simulink model "case5"  (R2024b)
settings: Solver=FixedStepAuto  StartTime=0  StopTime=1  FixedStep=1e-7  RelTol=1e-3
values from neighbouring files (symbols this model uses):
  SG_D_1_D = 0.01056    [IEEE9_case_parameters.m]    (also in case1_parameters.m; case2_parameters.m; case3_parameters.m; case4_parameters.m)
  SG_D_1_EnableSaturation = 0    [IEEE9_case_parameters.m]    (also in case1_parameters.m; case2_parameters.m; case3_parameters.m; case4_parameters.m)
  SG_D_1_f0 = 60    [IEEE9_case_parameters.m]    (also in case1_parameters.m; case2_parameters.m; case3_parameters.m; case4_parameters.m)
  SG_D_1_H = 7.5    [IEEE9_case_parameters.m]    (also in case1_parameters.m; case2_parameters.m; case3_parameters.m; case4_parameters.m)
  SG_D_1_K_A = 20    [IEEE9_case_parameters.m]    (also in case1_parameters.m; case2_parameters.m; case3_parameters.m; case4_parameters.m)
  SG_D_1_K_E = 1.000000e+1    (= 10)    [IEEE9_case_parameters.m]    (also in case1_parameters.m; case2_parameters.m; case3_parameters.m; case4_parameters.m)
  SG_D_1_K_F = 2.363    [IEEE9_case_parameters.m]    (also in case1_parameters.m; case2_parameters.m; case3_parameters.m; case4_parameters.m)
  SG_D_1_K_s = 0.5    [IEEE9_case_parameters.m]    (also in case1_parameters.m = 5; case2_parameters.m = 5; case3_parameters.m = 5; case4_parameters.m = 5)
  SG_D_1_R_a = 0.001088    [IEEE9_case_parameters.m]    (also in case1_parameters.m; case2_parameters.m; case3_parameters.m; case4_parameters.m)
  SG_D_1_S_A = 1    [IEEE9_case_parameters.m]    (also in case1_parameters.m; case2_parameters.m; case3_parameters.m; case4_parameters.m)
  SG_D_1_S_B = 0.103    [IEEE9_case_parameters.m]    (also in case1_parameters.m; case2_parameters.m; case3_parameters.m; case4_parameters.m)
  SG_D_1_S_N = 10.659857    [IEEE9_case_parameters.m]    (also in case1_parameters.m; case2_parameters.m; case3_parameters.m; case4_parameters.m)
  SG_D_1_SpeedPara = 200    [IEEE9_case_parameters.m]    (also in case1_parameters.m; case2_parameters.m; case3_parameters.m; case4_parameters.m)
  SG_D_1_T_0 = 0.720173    [IEEE9_case_parameters.m]    (also in case1_parameters.m = 0.755522; case2_parameters.m = 0.808931; case3_parameters.m = 0.869402; case4_parameters.m = 0.729316)
  SG_D_1_T_1 = 0.3    [IEEE9_case_parameters.m]    (also in case1_parameters.m; case2_parameters.m; case3_parameters.m; case4_parameters.m)
  SG_D_1_T_2 = 0.05    [IEEE9_case_parameters.m]    (also in case1_parameters.m; case2_parameters.m; case3_parameters.m; case4_parameters.m)
  SG_D_1_T_3 = 0.02    [IEEE9_case_parameters.m]    (also in case1_parameters.m; case2_parameters.m; case3_parameters.m; case4_parameters.m)
  SG_D_1_T_4 = 0.005    [IEEE9_case_parameters.m]    (also in case1_parameters.m; case2_parameters.m; case3_parameters.m; case4_parameters.m)
  SG_D_1_T_A = 0.02    [IEEE9_case_parameters.m]    (also in case1_parameters.m; case2_parameters.m; case3_parameters.m; case4_parameters.m)
  SG_D_1_T_dd = 8.000000e+0    (= 8)    [IEEE9_case_parameters.m]    (also in case1_parameters.m; case2_parameters.m; case3_parameters.m; case4_parameters.m)
  SG_D_1_T_ddd = 0.04    [IEEE9_case_parameters.m]    (also in case1_parameters.m; case2_parameters.m; case3_parameters.m; case4_parameters.m)
  SG_D_1_T_E = 0.314    [IEEE9_case_parameters.m]    (also in case1_parameters.m; case2_parameters.m; case3_parameters.m; case4_parameters.m)
  SG_D_1_T_F = 0.35    [IEEE9_case_parameters.m]    (also in case1_parameters.m; case2_parameters.m; case3_parameters.m; case4_parameters.m)
  SG_D_1_T_qd = 0.8    [IEEE9_case_parameters.m]    (also in case1_parameters.m; case2_parameters.m; case3_parameters.m; case4_parameters.m)
  SG_D_1_T_qdd = 0.02    [IEEE9_case_parameters.m]    (also in case1_parameters.m; case2_parameters.m; case3_parameters.m; case4_parameters.m)
  SG_D_1_T_speed = 0.1    [IEEE9_case_parameters.m]    (also in case1_parameters.m = 200; case2_parameters.m = 200; case3_parameters.m = 200; case4_parameters.m = 200)
  SG_D_1_T_w = 0.5    [IEEE9_case_parameters.m]    (also in case1_parameters.m; case2_parameters.m; case3_parameters.m; case4_parameters.m)
  SG_D_1_V_ref = 1.990276    [IEEE9_case_parameters.m]    (also in case1_parameters.m = 2.042296; case2_parameters.m = 2.051388; case3_parameters.m = 2.089584; case4_parameters.m = 2.01845)
  SG_D_1_w_ref = 376.991118    [IEEE9_case_parameters.m]    (also in case1_parameters.m; case2_parameters.m; case3_parameters.m; case4_parameters.m)
  SG_D_1_wb = 6.000000e+1    (= 60)    [IEEE9_case_parameters.m]    (also in case1_parameters.m; case2_parameters.m; case3_parameters.m; case4_parameters.m)
  SG_D_1_x_d = 1.9    [IEEE9_case_parameters.m]    (also in case1_parameters.m; case2_parameters.m; case3_parameters.m; case4_parameters.m)
  SG_D_1_x_dd = 0.302    [IEEE9_case_parameters.m]    (also in case1_parameters.m; case2_parameters.m; case3_parameters.m; case4_parameters.m)
  SG_D_1_x_ddd = 0.204    [IEEE9_case_parameters.m]    (also in case1_parameters.m; case2_parameters.m; case3_parameters.m; case4_parameters.m)
  SG_D_1_x_l = 0.05    [IEEE9_case_parameters.m]    (also in case1_parameters.m; case2_parameters.m; case3_parameters.m; case4_parameters.m)
  SG_D_1_x_q = 1.3    [IEEE9_case_parameters.m]    (also in case1_parameters.m; case2_parameters.m; case3_parameters.m; case4_parameters.m)
  SG_D_1_x_qd = 0.5    [IEEE9_case_parameters.m]    (also in case1_parameters.m; case2_parameters.m; case3_parameters.m; case4_parameters.m)
  SG_D_1_x_qdd = 0.3    [IEEE9_case_parameters.m]    (also in case1_parameters.m; case2_parameters.m; case3_parameters.m; case4_parameters.m)
  SG_D_2_D = 0.02    [IEEE9_case_parameters.m]    (also in case1_parameters.m; case2_parameters.m; case3_parameters.m; case4_parameters.m)
  SG_D_2_EnableSaturation = 0    [IEEE9_case_parameters.m]    (also in case1_parameters.m; case2_parameters.m; case3_parameters.m; case4_parameters.m)
  SG_D_2_f0 = 60    [IEEE9_case_parameters.m]    (also in case1_parameters.m; case2_parameters.m; case3_parameters.m; case4_parameters.m)
  SG_D_2_H = 8.000000e+0    (= 8)    [IEEE9_case_parameters.m]    (also in case1_parameters.m; case2_parameters.m; case3_parameters.m; case4_parameters.m)
  SG_D_2_K_A = 20    [IEEE9_case_parameters.m]    (also in case1_parameters.m; case2_parameters.m; case3_parameters.m; case4_parameters.m)
  SG_D_2_K_E = 1.000000e+1    (= 10)    [IEEE9_case_parameters.m]    (also in case1_parameters.m; case2_parameters.m; case3_parameters.m; case4_parameters.m)
  SG_D_2_K_F = 2.363    [IEEE9_case_parameters.m]    (also in case1_parameters.m; case2_parameters.m; case3_parameters.m; case4_parameters.m)
  SG_D_2_K_s = 0.5    [IEEE9_case_parameters.m]    (also in case1_parameters.m = 4; case2_parameters.m = 4; case3_parameters.m = 4; case4_parameters.m = 4)
  SG_D_2_R_a = 0.001088    [IEEE9_case_parameters.m]    (also in case1_parameters.m; case2_parameters.m; case3_parameters.m; case4_parameters.m)
  SG_D_2_S_A = 1    [IEEE9_case_parameters.m]    (also in case1_parameters.m; case2_parameters.m; case3_parameters.m; case4_parameters.m)
  SG_D_2_S_B = 0.103    [IEEE9_case_parameters.m]    (also in case1_parameters.m; case2_parameters.m; case3_parameters.m; case4_parameters.m)
  SG_D_2_S_N = 10.659857    [IEEE9_case_parameters.m]    (also in case1_parameters.m; case2_parameters.m; case3_parameters.m; case4_parameters.m)
  SG_D_2_SpeedPara = 200    [IEEE9_case_parameters.m]    (also in case1_parameters.m; case2_parameters.m; case3_parameters.m; case4_parameters.m)
  SG_D_2_T_0 = 1.632913    [IEEE9_case_parameters.m]    (also in case1_parameters.m = 1.632925; case2_parameters.m = 1.632915; case3_parameters.m = 1.632914; case4_parameters.m = 1.632927)
  SG_D_2_T_1 = 0.2    [IEEE9_case_parameters.m]    (also in case1_parameters.m; case2_parameters.m; case3_parameters.m; case4_parameters.m)
  SG_D_2_T_2 = 0.05    [IEEE9_case_parameters.m]    (also in case1_parameters.m; case2_parameters.m; case3_parameters.m; case4_parameters.m)
  SG_D_2_T_3 = 0.02    [IEEE9_case_parameters.m]    (also in case1_parameters.m; case2_parameters.m; case3_parameters.m; case4_parameters.m)
  SG_D_2_T_4 = 0.005    [IEEE9_case_parameters.m]    (also in case1_parameters.m; case2_parameters.m; case3_parameters.m; case4_parameters.m)
  SG_D_2_T_A = 0.02    [IEEE9_case_parameters.m]    (also in case1_parameters.m; case2_parameters.m; case3_parameters.m; case4_parameters.m)
  SG_D_2_T_dd = 7.9    [IEEE9_case_parameters.m]    (also in case1_parameters.m; case2_parameters.m; case3_parameters.m; case4_parameters.m)
  SG_D_2_T_ddd = 0.04    [IEEE9_case_parameters.m]    (also in case1_parameters.m; case2_parameters.m; case3_parameters.m; case4_parameters.m)
  SG_D_2_T_E = 0.314    [IEEE9_case_parameters.m]    (also in case1_parameters.m; case2_parameters.m; case3_parameters.m; case4_parameters.m)
  SG_D_2_T_F = 0.35    [IEEE9_case_parameters.m]    (also in case1_parameters.m; case2_parameters.m; case3_parameters.m; case4_parameters.m)
  SG_D_2_T_qd = 0.8    [IEEE9_case_parameters.m]    (also in case1_parameters.m; case2_parameters.m; case3_parameters.m; case4_parameters.m)
  SG_D_2_T_qdd = 0.015    [IEEE9_case_parameters.m]    (also in case1_parameters.m; case2_parameters.m; case3_parameters.m; case4_parameters.m)
  SG_D_2_T_speed = 0.1    [IEEE9_case_parameters.m]    (also in case1_parameters.m = 150; case2_parameters.m = 150; case3_parameters.m = 150; case4_parameters.m = 150)
  SG_D_2_T_w = 0.35    [IEEE9_case_parameters.m]    (also in case1_parameters.m; case2_parameters.m; case3_parameters.m; case4_parameters.m)
  SG_D_2_V_ref = 2.58547    [IEEE9_case_parameters.m]    (also in case1_parameters.m = 2.597896; case2_parameters.m = 2.587136; case3_parameters.m = 2.586042; case4_parameters.m = 2.599679)
  SG_D_2_w_ref = 376.991118    [IEEE9_case_parameters.m]    (also in case1_parameters.m; case2_parameters.m; case3_parameters.m; case4_parameters.m)
  SG_D_2_wb = 6.000000e+1    (= 60)    [IEEE9_case_parameters.m]    (also in case1_parameters.m; case2_parameters.m; case3_parameters.m; case4_parameters.m)
  SG_D_2_x_d = 1.8    [IEEE9_case_parameters.m]    (also in case1_parameters.m; case2_parameters.m; case3_parameters.m; case4_parameters.m)
  SG_D_2_x_dd = 0.302    [IEEE9_case_parameters.m]    (also in case1_parameters.m; case2_parameters.m; case3_parameters.m; case4_parameters.m)
  SG_D_2_x_ddd = 0.204    [IEEE9_case_parameters.m]    (also in case1_parameters.m; case2_parameters.m; case3_parameters.m; case4_parameters.m)
  SG_D_2_x_l = 0.05    [IEEE9_case_parameters.m]    (also in case1_parameters.m; case2_parameters.m; case3_parameters.m; case4_parameters.m)
  SG_D_2_x_q = 1.25    [IEEE9_case_parameters.m]    (also in case1_parameters.m; case2_parameters.m; case3_parameters.m; case4_parameters.m)
  SG_D_2_x_qd = 0.5    [IEEE9_case_parameters.m]    (also in case1_parameters.m; case2_parameters.m; case3_parameters.m; case4_parameters.m)
  SG_D_2_x_qdd = 0.3    [IEEE9_case_parameters.m]    (also in case1_parameters.m; case2_parameters.m; case3_parameters.m; case4_parameters.m)
  SG_D_3_D = 0.02    [IEEE9_case_parameters.m]    (also in case1_parameters.m; case2_parameters.m; case3_parameters.m; case4_parameters.m)
  SG_D_3_EnableSaturation = 0    [IEEE9_case_parameters.m]    (also in case1_parameters.m; case2_parameters.m; case3_parameters.m; case4_parameters.m)
  SG_D_3_f0 = 60    [IEEE9_case_parameters.m]    (also in case1_parameters.m; case2_parameters.m; case3_parameters.m; case4_parameters.m)
  SG_D_3_H = 7.7    [IEEE9_case_parameters.m]    (also in case1_parameters.m; case2_parameters.m; case3_parameters.m; case4_parameters.m)
  SG_D_3_K_A = 20    [IEEE9_case_parameters.m]    (also in case1_parameters.m; case2_parameters.m; case3_parameters.m; case4_parameters.m)
  SG_D_3_K_E = 1.000000e+1    (= 10)    [IEEE9_case_parameters.m]    (also in case1_parameters.m; case2_parameters.m; case3_parameters.m; case4_parameters.m)
  SG_D_3_K_F = 2.363    [IEEE9_case_parameters.m]    (also in case1_parameters.m; case2_parameters.m; case3_parameters.m; case4_parameters.m)
  SG_D_3_K_s = 0.2    [IEEE9_case_parameters.m]    (also in case1_parameters.m = 2; case2_parameters.m = 2; case3_parameters.m = 2; case4_parameters.m = 2)
  SG_D_3_R_a = 0.001088    [IEEE9_case_parameters.m]    (also in case1_parameters.m; case2_parameters.m; case3_parameters.m; case4_parameters.m)
  SG_D_3_S_A = 1    [IEEE9_case_parameters.m]    (also in case1_parameters.m; case2_parameters.m; case3_parameters.m; case4_parameters.m)
  SG_D_3_S_B = 0.103    [IEEE9_case_parameters.m]    (also in case1_parameters.m; case2_parameters.m; case3_parameters.m; case4_parameters.m)
  SG_D_3_S_N = 10.659857    [IEEE9_case_parameters.m]    (also in case1_parameters.m; case2_parameters.m; case3_parameters.m; case4_parameters.m)
  SG_D_3_SpeedPara = 200    [IEEE9_case_parameters.m]    (also in case1_parameters.m; case2_parameters.m; case3_parameters.m; case4_parameters.m)
  SG_D_3_T_0 = 0.850788    [IEEE9_case_parameters.m]    (also in case1_parameters.m = 0.850786; case2_parameters.m = 0.850787; case3_parameters.m; case4_parameters.m = 0.850786)
  SG_D_3_T_1 = 0.2    [IEEE9_case_parameters.m]    (also in case1_parameters.m; case2_parameters.m; case3_parameters.m; case4_parameters.m)
  SG_D_3_T_2 = 0.05    [IEEE9_case_parameters.m]    (also in case1_parameters.m; case2_parameters.m; case3_parameters.m; case4_parameters.m)
  SG_D_3_T_3 = 0.02    [IEEE9_case_parameters.m]    (also in case1_parameters.m; case2_parameters.m; case3_parameters.m; case4_parameters.m)
  SG_D_3_T_4 = 0.005    [IEEE9_case_parameters.m]    (also in case1_parameters.m; case2_parameters.m; case3_parameters.m; case4_parameters.m)
  SG_D_3_T_A = 0.02    [IEEE9_case_parameters.m]    (also in case1_parameters.m; case2_parameters.m; case3_parameters.m; case4_parameters.m)
  SG_D_3_T_dd = 8.1    [IEEE9_case_parameters.m]    (also in case1_parameters.m; case2_parameters.m; case3_parameters.m; case4_parameters.m)
  SG_D_3_T_ddd = 0.04    [IEEE9_case_parameters.m]    (also in case1_parameters.m; case2_parameters.m; case3_parameters.m; case4_parameters.m)
  SG_D_3_T_E = 0.314    [IEEE9_case_parameters.m]    (also in case1_parameters.m; case2_parameters.m; case3_parameters.m; case4_parameters.m)
  SG_D_3_T_F = 0.35    [IEEE9_case_parameters.m]    (also in case1_parameters.m; case2_parameters.m; case3_parameters.m; case4_parameters.m)
  SG_D_3_T_qd = 0.8    [IEEE9_case_parameters.m]    (also in case1_parameters.m; case2_parameters.m; case3_parameters.m; case4_parameters.m)
  SG_D_3_T_qdd = 0.015    [IEEE9_case_parameters.m]    (also in case1_parameters.m; case2_parameters.m; case3_parameters.m; case4_parameters.m)
  SG_D_3_T_speed = 0.1    [IEEE9_case_parameters.m]    (also in case1_parameters.m = 180; case2_parameters.m = 180; case3_parameters.m = 180; case4_parameters.m = 180)
  SG_D_3_T_w = 0.4    [IEEE9_case_parameters.m]    (also in case1_parameters.m; case2_parameters.m; case3_parameters.m; case4_parameters.m)
  SG_D_3_V_ref = 1.892727    [IEEE9_case_parameters.m]    (also in case1_parameters.m = 1.906439; case2_parameters.m = 1.895535; case3_parameters.m = 1.892105; case4_parameters.m = 1.906598)
  SG_D_3_w_ref = 376.991118    [IEEE9_case_parameters.m]    (also in case1_parameters.m; case2_parameters.m; case3_parameters.m; case4_parameters.m)
  SG_D_3_wb = 6.000000e+1    (= 60)    [IEEE9_case_parameters.m]    (also in case1_parameters.m; case2_parameters.m; case3_parameters.m; case4_parameters.m)
  SG_D_3_x_d = 1.85    [IEEE9_case_parameters.m]    (also in case1_parameters.m; case2_parameters.m; case3_parameters.m; case4_parameters.m)
  SG_D_3_x_dd = 0.302    [IEEE9_case_parameters.m]    (also in case1_parameters.m; case2_parameters.m; case3_parameters.m; case4_parameters.m)
  SG_D_3_x_ddd = 0.204    [IEEE9_case_parameters.m]    (also in case1_parameters.m; case2_parameters.m; case3_parameters.m; case4_parameters.m)
  SG_D_3_x_l = 0.05    [IEEE9_case_parameters.m]    (also in case1_parameters.m; case2_parameters.m; case3_parameters.m; case4_parameters.m)
  SG_D_3_x_q = 1.2    [IEEE9_case_parameters.m]    (also in case1_parameters.m; case2_parameters.m; case3_parameters.m; case4_parameters.m)
  SG_D_3_x_qd = 0.5    [IEEE9_case_parameters.m]    (also in case1_parameters.m; case2_parameters.m; case3_parameters.m; case4_parameters.m)
  SG_D_3_x_qdd = 0.3    [IEEE9_case_parameters.m]    (also in case1_parameters.m; case2_parameters.m; case3_parameters.m; case4_parameters.m)
(part 10 of 12)

== system case5/SG_D_3/d_R_f_SG_D_3_block ==
  note: d_R_f_SG_D_3 in case5
      | $-\frac{R_{f,\mathrm{SG},D,3}-\frac{E_{\mathrm{fd},\mathrm{SG},D,3}\,K_{F}}{T_{F}}}{T_{F}}$
      | Automatically generated on 2025-10-31 19:13:03 .
  State_E_fd_SG_D_3_8b5d7 : Inport
  State_R_f_SG_D_3_2ac4f : Inport  Port=2
  Constant_K_F_e3408 : Constant  Value=K_F
  Constant_T_F_8f28c : Constant  Value=T_F
  Constant_T_F_f3a7a : Constant  Value=T_F
  Divide_cdbe2 : Product  Inputs=*/
  Divide_fd0b4 : Product  Inputs=*/
  Product_cf118 : Product
  Subtract_30a77 : Sum  Inputs=+-
  Blockout_d_R_f_SG_D_3_894a9 : Outport
  wires:
  State_E_fd_SG_D_3_8b5d7/1 -> Product_cf118/1
  Constant_T_F_8f28c/1 -> Divide_fd0b4/2
  Constant_K_F_e3408/1 -> Product_cf118/2
  Product_cf118/1 -> Divide_fd0b4/1
  Divide_fd0b4/1 -> Subtract_30a77/1
  State_R_f_SG_D_3_2ac4f/1 -> Subtract_30a77/2
  Subtract_30a77/1 -> Divide_cdbe2/1
  Constant_T_F_f3a7a/1 -> Divide_cdbe2/2
  Divide_cdbe2/1 -> Blockout_d_R_f_SG_D_3_894a9/1

== system case5/SG_D_3/d_T_m_SG_D_3_block ==
  note: d_T_m_SG_D_3 in case5
      | $-\frac{T_{m,\mathrm{SG},D,3}-T_{0}+\frac{\mathrm{SpeedPara}\,\left(w_{\mathrm{SG},D,3}-w_{\mathrm{ref}}\right)}{2\,f_{0}\,\pi }}{T_{\mathrm{speed}}}$
      | Automatically generated on 2025-10-31 19:12:52 .
  State_w_SG_D_3_0ca8a : Inport
  State_T_m_SG_D_3_db6e5 : Inport  Port=2
  Add_3c72c : Sum
  Add_817cc : Sum
  Constant_-1_34284 : Constant  Value=-1
  Constant_2.0_b08ac : Constant  Value=2.0
  Constant_SpeedPara_1be1d : Constant  Value=SpeedPara
  Constant_T_0_6266c : Constant  Value=T_0
  Constant_T_speed_5b405 : Constant  Value=T_speed
  Constant_f0_e0ee2 : Constant  Value=f0
  Constant_pi_6c19b : Constant  Value=pi
  Constant_w_ref_8af40 : Constant  Value=w_ref
  Divide_7f5c9 : Product  Inputs=*/
  Divide_c0706 : Product  Inputs=*/
  Product_5f391 : Product
  Product_62ec6 : Product
  Product_a0b65 : Product
  Product_d16a5 : Product
  Subtract_61ee2 : Sum  Inputs=+-
  Blockout_d_T_m_SG_D_3_d3830 : Outport
  wires:
  Constant_SpeedPara_1be1d/1 -> Product_5f391/1
  Constant_-1_34284/1 -> Product_d16a5/1
  Constant_w_ref_8af40/1 -> Add_817cc/2
  State_w_SG_D_3_0ca8a/1 -> Product_d16a5/2
  Constant_2.0_b08ac/1 -> Product_62ec6/1
  Product_d16a5/1 -> Add_817cc/1
  Constant_pi_6c19b/1 -> Product_62ec6/2
  Add_817cc/1 -> Product_5f391/2
  Product_62ec6/1 -> Product_a0b65/1
  Constant_f0_e0ee2/1 -> Product_a0b65/2
  Product_5f391/1 -> Divide_c0706/1
  Product_a0b65/1 -> Divide_c0706/2
  Divide_c0706/1 -> Add_3c72c/1
  Constant_T_0_6266c/1 -> Add_3c72c/2
  Add_3c72c/1 -> Subtract_61ee2/1
  State_T_m_SG_D_3_db6e5/1 -> Subtract_61ee2/2
  Subtract_61ee2/1 -> Divide_7f5c9/1
  Constant_T_speed_5b405/1 -> Divide_7f5c9/2
  Divide_7f5c9/1 -> Blockout_d_T_m_SG_D_3_d3830/1

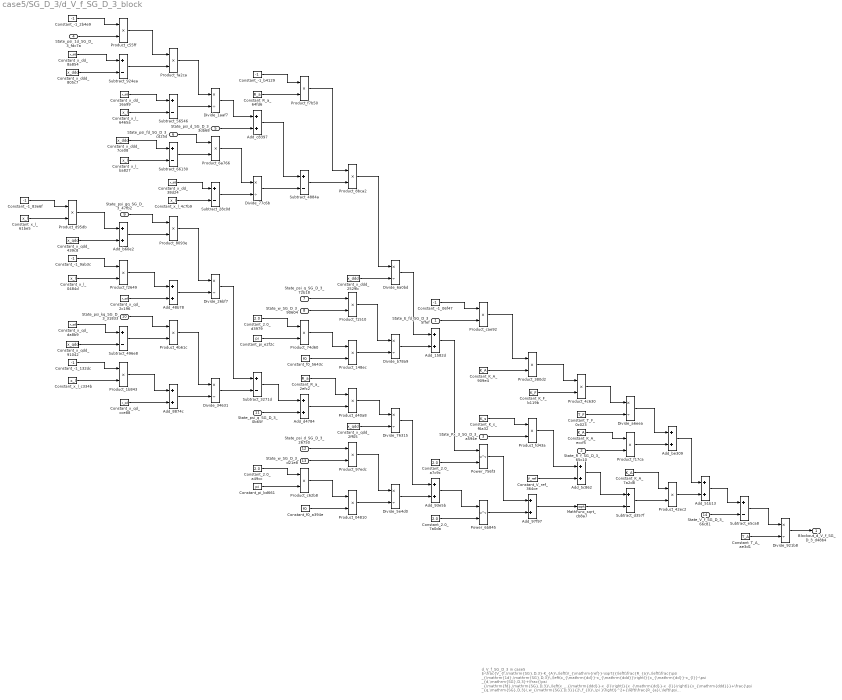
== system case5/SG_D_3/d_V_f_SG_D_3_block ==
  note: d_V_f_SG_D_3 in case5
      | $-\frac{V_{f,\mathrm{SG},D,3}-K_{A}\,\left(V_{\mathrm{ref}}-\sqrt{{\left(\frac{R_{a}\,\left(\frac{\psi _{\mathrm{1d},\mathrm{SG},D,3}\,\left(x_{\mathrm{dd}}-x_{\mathrm{ddd}}\right)}{x_{\mathrm{dd}}-x_{l}}-\psi _{d,\mathrm{SG},D,3}+\frac{\psi _{\mathrm{fd},\mathrm{SG},D,3}\,\left(x_{\mathrm{ddd}}-x_{l}\right)}{x_{\mathrm{dd}}-x_{l}}\right)}{x_{\mathrm{ddd}}}+\frac{\psi _{q,\mathrm{SG},D,3}\,w_{\mathrm{SG},D,3}}{2\,f_{0}\,\pi }\right)}^2+{\left(\frac{R_{a}\,\left(\psi _{q,\mathrm{SG},D,3}+\frac{\psi _{\mathrm{gq},\mathrm{SG},D,3}\,\left(x_{l}-x_{\mathrm{qdd}}\right)}{x_{l}-x_{\mathrm{qd}}}+\frac{\psi _{\mathrm{kq},\mathrm{SG},D,3}\,\left(x_{\mathrm{qd}}-x_{\mathrm{qdd}}\right)}{x_{l}-x_{\mathrm{qd}}}\right)}{x_{\mathrm{qdd}}}+\frac{\psi _{d,\mathrm{SG},D,3}\,w_{\mathrm{SG},D,3}}{2\,f_{0}\,\pi }\right)}^2}+K_{s}\,\mathrm{Px}_{3,\mathrm{SG},D,3}\right)-K_{A}\,R_{f,\mathrm{SG},D,3}+\frac{E_{\mathrm{fd},\mathrm{SG},D,3}\,K_{A}\,K_{F}}{T_{F}}}{T_{A}}$
      | Automatically generated on 2025-10-31 19:13:01 .
  State_E_fd_SG_D_3_5ffef : Inport
  State_R_f_SG_D_3_65c10 : Inport  Port=2
  State_Px_3_SG_D_3_a594e : Inport  Port=3
  State_psi_1d_SG_D_3_fdc7a : Inport  Port=4
  State_psi_d_SG_D_3_3db68 : Inport  Port=5
  State_psi_fd_SG_D_3_cd25d : Inport  Port=6
  State_psi_q_SG_D_3_72b18 : Inport  Port=7
  State_w_SG_D_3_90604 : Inport  Port=8
  State_psi_gq_SG_D_3_47fb2 : Inport  Port=9
  State_psi_kq_SG_D_3_31833 : Inport  Port=10
  State_psi_q_SG_D_3_0b65f : Inport  Port=11
  State_psi_d_SG_D_3_26750 : Inport  Port=12
  State_w_SG_D_3_d21e8 : Inport  Port=13
  State_V_f_SG_D_3_66c81 : Inport  Port=14
  Add_1582d : Sum
  Add_48b78 : Sum
  Add_51b13 : Sum
  Add_5c862 : Sum
  Add_8874c : Sum
  Add_93e5b : Sum
  Add_97f97 : Sum
  Add_b60e2 : Sum
  Add_be309 : Sum
  Add_c8397 : Sum
  Add_d4784 : Sum
  Constant_-1_06f47 : Constant  Value=-1
  Constant_-1_132dc : Constant  Value=-1
  Constant_-1_2b4e9 : Constant  Value=-1
  Constant_-1_83e6f : Constant  Value=-1
  Constant_-1_9ab3c : Constant  Value=-1
  Constant_-1_b4129 : Constant  Value=-1
  Constant_2.0_7a0da : Constant  Value=2.0
  Constant_2.0_a49cc : Constant  Value=2.0
  Constant_2.0_a7c9c : Constant  Value=2.0
  Constant_2.0_d3979 : Constant  Value=2.0
  Constant_K_A_7a2d8 : Constant  Value=K_A
  Constant_K_A_909e4 : Constant  Value=K_A
  Constant_K_A_eccf5 : Constant  Value=K_A
  Constant_K_F_b119b : Constant  Value=K_F
  Constant_K_s_f6a32 : Constant  Value=K_s
  Constant_R_a_2efc2 : Constant  Value=R_a
  Constant_R_a_64fd6 : Constant  Value=R_a
  Constant_T_A_ae3d1 : Constant  Value=T_A
  Constant_T_F_0c023 : Constant  Value=T_F
  Constant_V_ref_364ce : Constant  Value=V_ref
  Constant_f0_5643c : Constant  Value=f0
  Constant_f0_a394e : Constant  Value=f0
  Constant_pi_bd661 : Constant  Value=pi
  Constant_pi_e2f2c : Constant  Value=pi
  Constant_x_dd_16a99 : Constant  Value=x_dd
  Constant_x_dd_38d24 : Constant  Value=x_dd
  Constant_x_dd_8a854 : Constant  Value=x_dd
  Constant_x_ddd_2529b : Constant  Value=x_ddd
  Constant_x_ddd_7ce08 : Constant  Value=x_ddd
  Constant_x_ddd_805c7 : Constant  Value=x_ddd
  Constant_x_l_0484d : Constant  Value=x_l
  Constant_x_l_4c7b9 : Constant  Value=x_l
  Constant_x_l_61be5 : Constant  Value=x_l
  Constant_x_l_6465a : Constant  Value=x_l
  Constant_x_l_ba827 : Constant  Value=x_l
  Constant_x_l_c334b : Constant  Value=x_l
  Constant_x_qd_2c196 : Constant  Value=x_qd
  Constant_x_qd_cce88 : Constant  Value=x_qd
  Constant_x_qd_da8b9 : Constant  Value=x_qd
  Constant_x_qdd_2ff05 : Constant  Value=x_qdd
  Constant_x_qdd_439c8 : Constant  Value=x_qdd
  Constant_x_qdd_91042 : Constant  Value=x_qdd
  Divide_1aaf7 : Product  Inputs=*/
  Divide_26bf7 : Product  Inputs=*/
  Divide_34631 : Product  Inputs=*/
  Divide_5e4d0 : Product  Inputs=*/
  Divide_6a0bd : Product  Inputs=*/
  Divide_76315 : Product  Inputs=*/
  Divide_77c6b : Product  Inputs=*/
  Divide_921b8 : Product  Inputs=*/
  Divide_a6eea : Product  Inputs=*/
  Divide_b78a9 : Product  Inputs=*/
  MathFunc_sqrt_cb8a7 : Sqrt
  Power_6b845 : Math  Operator=pow
  Power_756f3 : Math  Operator=pow
  Product_04810 : Product
  Product_148ec : Product
  Product_1b843 : Product
  Product_380d2 : Product
  Product_42ec2 : Product
  Product_4b61c : Product
  Product_4c630 : Product
  Product_6a766 : Product
  Product_74d60 : Product
  Product_8093e : Product
  Product_8bca2 : Product
  Product_97edc : Product
  Product_c55ff : Product
  Product_c62b8 : Product
  Product_cae92 : Product
  Product_d40a8 : Product
  Product_d95db : Product
  Product_f1510 : Product
  Product_f17ca : Product
  Product_f2649 : Product
  Product_f7b50 : Product
  Product_fa2ca : Product
  Product_fd43a : Product
  Subtract_28c0d : Sum  Inputs=+-
  Subtract_3271d : Sum  Inputs=+-
  Subtract_4884a : Sum  Inputs=+-
  Subtract_496e8 : Sum  Inputs=+-
  Subtract_56546 : Sum  Inputs=+-
  Subtract_66130 : Sum  Inputs=+-
  Subtract_924ea : Sum  Inputs=+-
  Subtract_d357f : Sum  Inputs=+-
  Subtract_e5ca8 : Sum  Inputs=+-
  Blockout_d_V_f_SG_D_3_d48b4 : Outport
  wires:
  Constant_K_A_eccf5/1 -> Product_f17ca/1
  Constant_-1_83e6f/1 -> Product_d95db/1
  Subtract_66130/1 -> Product_6a766/2
  Constant_x_l_61be5/1 -> Product_d95db/2
  Divide_5e4d0/1 -> Add_93e5b/2
  Constant_-1_2b4e9/1 -> Product_c55ff/1
  State_psi_1d_SG_D_3_fdc7a/1 -> Product_c55ff/2
  Constant_x_dd_8a854/1 -> Subtract_924ea/1
  Divide_77c6b/1 -> Subtract_4884a/2
  Product_d95db/1 -> Add_b60e2/1
  Constant_x_qdd_439c8/1 -> Add_b60e2/2
  Constant_x_ddd_805c7/1 -> Subtract_924ea/2
  Constant_2.0_7a0da/1 -> Power_6b845/2
  Constant_-1_9ab3c/1 -> Product_f2649/1
  Divide_26bf7/1 -> Subtract_3271d/1
  Subtract_56546/1 -> Divide_1aaf7/2
  Constant_x_l_0484d/1 -> Product_f2649/2
  Constant_x_qd_da8b9/1 -> Subtract_496e8/1
  State_w_SG_D_3_90604/1 -> Product_f1510/2
  Constant_x_qdd_91042/1 -> Subtract_496e8/2
  Constant_2.0_d3979/1 -> Product_74d60/1
  Constant_-1_132dc/1 -> Product_1b843/1
  Constant_pi_e2f2c/1 -> Product_74d60/2
  Add_c8397/1 -> Subtract_4884a/1
  Constant_x_l_c334b/1 -> Product_1b843/2
  Product_c55ff/1 -> Product_fa2ca/1
  Subtract_924ea/1 -> Product_fa2ca/2
  Constant_2.0_a49cc/1 -> Product_c62b8/1
  Constant_x_dd_16a99/1 -> Subtract_56546/1
  Constant_pi_bd661/1 -> Product_c62b8/2
  Constant_x_l_6465a/1 -> Subtract_56546/2
  Constant_x_ddd_7ce08/1 -> Subtract_66130/1
  Constant_x_l_ba827/1 -> Subtract_66130/2
  State_psi_gq_SG_D_3_47fb2/1 -> Product_8093e/1
  Constant_x_l_4c7b9/1 -> Subtract_28c0d/2
  Add_b60e2/1 -> Product_8093e/2
  Product_f2649/1 -> Add_48b78/1
  Product_8093e/1 -> Divide_26bf7/1
  Constant_x_qd_2c196/1 -> Add_48b78/2
  State_psi_kq_SG_D_3_31833/1 -> Product_4b61c/1
  State_psi_q_SG_D_3_72b18/1 -> Product_f1510/1
  Add_1582d/1 -> Power_756f3/1
  Subtract_496e8/1 -> Product_4b61c/2
  Constant_f0_5643c/1 -> Product_148ec/2
  Product_74d60/1 -> Product_148ec/1
  Constant_x_qd_cce88/1 -> Add_8874c/2
  Product_1b843/1 -> Add_8874c/1
  Product_fa2ca/1 -> Divide_1aaf7/1
  State_psi_fd_SG_D_3_cd25d/1 -> Product_6a766/1
  Constant_x_dd_38d24/1 -> Subtract_28c0d/1
  Add_48b78/1 -> Divide_26bf7/2
  Add_97f97/1 -> MathFunc_sqrt_cb8a7/1
  Product_4b61c/1 -> Divide_34631/1
  Add_8874c/1 -> Divide_34631/2
  Product_f7b50/1 -> Product_8bca2/1
  Divide_1aaf7/1 -> Add_c8397/1
  Add_5c862/1 -> Subtract_d357f/1
  State_psi_d_SG_D_3_3db68/1 -> Add_c8397/2
  Product_6a766/1 -> Divide_77c6b/1
  Subtract_28c0d/1 -> Divide_77c6b/2
  MathFunc_sqrt_cb8a7/1 -> Subtract_d357f/2
  Divide_34631/1 -> Subtract_3271d/2
  Constant_-1_b4129/1 -> Product_f7b50/1
  Constant_R_a_64fd6/1 -> Product_f7b50/2
  Subtract_3271d/1 -> Add_d4784/1
  State_psi_q_SG_D_3_0b65f/1 -> Add_d4784/2
  Subtract_4884a/1 -> Product_8bca2/2
  Constant_R_a_2efc2/1 -> Product_d40a8/1
  Add_d4784/1 -> Product_d40a8/2
  State_psi_d_SG_D_3_26750/1 -> Product_97edc/1
  State_w_SG_D_3_d21e8/1 -> Product_97edc/2
  Product_c62b8/1 -> Product_04810/1
  Constant_f0_a394e/1 -> Product_04810/2
  Product_8bca2/1 -> Divide_6a0bd/1
  Constant_x_ddd_2529b/1 -> Divide_6a0bd/2
  Product_f1510/1 -> Divide_b78a9/1
  Product_148ec/1 -> Divide_b78a9/2
  Product_d40a8/1 -> Divide_76315/1
  Constant_x_qdd_2ff05/1 -> Divide_76315/2
  Product_97edc/1 -> Divide_5e4d0/1
  Product_04810/1 -> Divide_5e4d0/2
  Divide_6a0bd/1 -> Add_1582d/1
  Divide_b78a9/1 -> Add_1582d/2
  Divide_76315/1 -> Add_93e5b/1
  Constant_-1_06f47/1 -> Product_cae92/1
  State_E_fd_SG_D_3_5ffef/1 -> Product_cae92/2
  Constant_2.0_a7c9c/1 -> Power_756f3/2
  Add_93e5b/1 -> Power_6b845/1
  Product_cae92/1 -> Product_380d2/1
  Constant_K_A_909e4/1 -> Product_380d2/2
  Constant_K_s_f6a32/1 -> Product_fd43a/1
  State_Px_3_SG_D_3_a594e/1 -> Product_fd43a/2
  Power_756f3/1 -> Add_97f97/1
  Power_6b845/1 -> Add_97f97/2
  Product_380d2/1 -> Product_4c630/1
  Constant_K_F_b119b/1 -> Product_4c630/2
  Product_fd43a/1 -> Add_5c862/1
  Constant_V_ref_364ce/1 -> Add_5c862/2
  Product_4c630/1 -> Divide_a6eea/1
  Constant_T_F_0c023/1 -> Divide_a6eea/2
  Add_51b13/1 -> Subtract_e5ca8/1
  State_R_f_SG_D_3_65c10/1 -> Product_f17ca/2
  Divide_a6eea/1 -> Add_be309/1
  Product_f17ca/1 -> Add_be309/2
  Constant_K_A_7a2d8/1 -> Product_42ec2/1
  Subtract_d357f/1 -> Product_42ec2/2
  Add_be309/1 -> Add_51b13/1
  Product_42ec2/1 -> Add_51b13/2
  State_V_f_SG_D_3_66c81/1 -> Subtract_e5ca8/2
  Subtract_e5ca8/1 -> Divide_921b8/1
  Constant_T_A_ae3d1/1 -> Divide_921b8/2
  Divide_921b8/1 -> Blockout_d_V_f_SG_D_3_d48b4/1

== system case5/SG_D_3/d_psi_1d_SG_D_3_block ==
  note: d_psi_1d_SG_D_3 in case5
      | $-\frac{\psi _{\mathrm{1d},\mathrm{SG},D,3}-\psi _{\mathrm{fd},\mathrm{SG},D,3}+\frac{\left(x_{\mathrm{dd}}-x_{l}\right)\,\left(\frac{\psi _{\mathrm{1d},\mathrm{SG},D,3}\,\left(x_{\mathrm{dd}}-x_{\mathrm{ddd}}\right)}{x_{\mathrm{dd}}-x_{l}}-\psi _{d,\mathrm{SG},D,3}+\frac{\psi _{\mathrm{fd},\mathrm{SG},D,3}\,\left(x_{\mathrm{ddd}}-x_{l}\right)}{x_{\mathrm{dd}}-x_{l}}\right)}{x_{\mathrm{ddd}}}}{T_{\mathrm{ddd}}}$
      | Automatically generated on 2025-10-31 19:12:32 .
  State_psi_1d_SG_D_3_3b403 : Inport
  State_psi_fd_SG_D_3_f9b6a : Inport  Port=2
  State_psi_1d_SG_D_3_4c72e : Inport  Port=3
  State_psi_d_SG_D_3_3e3a9 : Inport  Port=4
  State_psi_fd_SG_D_3_649d9 : Inport  Port=5
  Add_0b0c8 : Sum
  Add_92af5 : Sum
  Add_95a06 : Sum
  Constant_-1_86e6d : Constant  Value=-1
  Constant_-1_d9768 : Constant  Value=-1
  Constant_T_ddd_6cba8 : Constant  Value=T_ddd
  Constant_x_dd_14902 : Constant  Value=x_dd
  Constant_x_dd_8d1e4 : Constant  Value=x_dd
  Constant_x_dd_a0af1 : Constant  Value=x_dd
  Constant_x_dd_c7e96 : Constant  Value=x_dd
  Constant_x_ddd_a8048 : Constant  Value=x_ddd
  Constant_x_ddd_ab569 : Constant  Value=x_ddd
  Constant_x_ddd_ec5c8 : Constant  Value=x_ddd
  Constant_x_l_4da59 : Constant  Value=x_l
  Constant_x_l_7793e : Constant  Value=x_l
  Constant_x_l_bc55c : Constant  Value=x_l
  Constant_x_l_f8aff : Constant  Value=x_l
  Divide_2aa39 : Product  Inputs=*/
  Divide_5bbe6 : Product  Inputs=*/
  Divide_9353d : Product  Inputs=*/
  Divide_ae151 : Product  Inputs=*/
  Product_3a034 : Product
  Product_90e82 : Product
  Product_a4db2 : Product
  Product_af1b4 : Product
  Product_b14b4 : Product
  Subtract_07ee1 : Sum  Inputs=+-
  Subtract_25af9 : Sum  Inputs=+-
  Subtract_2e957 : Sum  Inputs=+-
  Subtract_3ae9e : Sum  Inputs=+-
  Subtract_3dda6 : Sum  Inputs=+-
  Subtract_99ba5 : Sum  Inputs=+-
  Blockout_d_psi_1d_SG_D_3_0c79f : Outport
  wires:
  Divide_ae151/1 -> Add_92af5/1
  Subtract_3ae9e/1 -> Product_b14b4/2
  Constant_-1_86e6d/1 -> Product_a4db2/1
  Constant_x_dd_8d1e4/1 -> Subtract_25af9/1
  State_psi_1d_SG_D_3_4c72e/1 -> Product_a4db2/2
  Product_a4db2/1 -> Product_b14b4/1
  Constant_x_dd_a0af1/1 -> Subtract_3ae9e/1
  Constant_x_ddd_ec5c8/1 -> Subtract_3ae9e/2
  Constant_x_l_4da59/1 -> Subtract_25af9/2
  Constant_x_ddd_a8048/1 -> Subtract_2e957/1
  Divide_2aa39/1 -> Blockout_d_psi_1d_SG_D_3_0c79f/1
  Constant_x_l_bc55c/1 -> Subtract_2e957/2
  Product_b14b4/1 -> Divide_ae151/1
  Subtract_25af9/1 -> Divide_ae151/2
  State_psi_fd_SG_D_3_649d9/1 -> Product_3a034/1
  Subtract_2e957/1 -> Product_3a034/2
  Constant_x_dd_14902/1 -> Subtract_07ee1/1
  Constant_x_l_f8aff/1 -> Subtract_07ee1/2
  State_psi_d_SG_D_3_3e3a9/1 -> Add_92af5/2
  Product_3a034/1 -> Divide_5bbe6/1
  Subtract_07ee1/1 -> Divide_5bbe6/2
  Constant_x_dd_c7e96/1 -> Subtract_3dda6/1
  Constant_x_l_7793e/1 -> Subtract_3dda6/2
  Add_92af5/1 -> Subtract_99ba5/1
  Divide_5bbe6/1 -> Subtract_99ba5/2
  Constant_-1_d9768/1 -> Product_af1b4/1
  State_psi_1d_SG_D_3_3b403/1 -> Product_af1b4/2
  State_psi_fd_SG_D_3_f9b6a/1 -> Add_95a06/2
  Subtract_3dda6/1 -> Product_90e82/1
  Subtract_99ba5/1 -> Product_90e82/2
  Product_af1b4/1 -> Add_95a06/1
  Product_90e82/1 -> Divide_9353d/1
  Constant_x_ddd_ab569/1 -> Divide_9353d/2
  Add_95a06/1 -> Add_0b0c8/1
  Divide_9353d/1 -> Add_0b0c8/2
  Add_0b0c8/1 -> Divide_2aa39/1
  Constant_T_ddd_6cba8/1 -> Divide_2aa39/2

== system case5/SG_D_3/d_psi_d_SG_D_3_block ==
  note: d_psi_d_SG_D_3 in case5
      | $2\,\pi \,f_{0}\,\left(v_{d,\mathrm{SG},D,3}\,\sin\left(\theta _{\mathrm{SG},D,3}\right)-v_{q,\mathrm{SG},D,3}\,\cos\left(\theta _{\mathrm{SG},D,3}\right)+\frac{R_{a}\,\left(\frac{\psi _{\mathrm{1d},\mathrm{SG},D,3}\,\left(x_{\mathrm{dd}}-x_{\mathrm{ddd}}\right)}{x_{\mathrm{dd}}-x_{l}}-\psi _{d,\mathrm{SG},D,3}+\frac{\psi _{\mathrm{fd},\mathrm{SG},D,3}\,\left(x_{\mathrm{ddd}}-x_{l}\right)}{x_{\mathrm{dd}}-x_{l}}\right)}{x_{\mathrm{ddd}}}+\frac{\psi _{q,\mathrm{SG},D,3}\,w_{\mathrm{SG},D,3}}{2\,f_{0}\,\pi }\right)$
      | Automatically generated on 2025-10-31 19:12:16 .
  State_psi_1d_SG_D_3_2013b : Inport
  State_psi_d_SG_D_3_d393d : Inport  Port=2
  State_psi_fd_SG_D_3_0e180 : Inport  Port=3
  Input_v_d_SG_D_3_606f6 : Inport  Port=4
  State_theta_SG_D_3_c5e42 : Inport  Port=5
  Input_v_q_SG_D_3_a4294 : Inport  Port=6
  State_theta_SG_D_3_aedc7 : Inport  Port=7
  State_psi_q_SG_D_3_01c82 : Inport  Port=8
  State_w_SG_D_3_5916e : Inport  Port=9
  Add_6de8d : Sum
  Add_95d2d : Sum
  Constant_-1_4ed88 : Constant  Value=-1
  Constant_-2.0_f1148 : Constant  Value=-2.0
  Constant_2.0_62dc7 : Constant  Value=2.0
  Constant_R_a_63c0e : Constant  Value=R_a
  Constant_f0_8dd7f : Constant  Value=f0
  Constant_f0_938aa : Constant  Value=f0
  Constant_pi_2a548 : Constant  Value=pi
  Constant_pi_3c9f0 : Constant  Value=pi
  Constant_x_dd_079ee : Constant  Value=x_dd
  Constant_x_dd_24fcc : Constant  Value=x_dd
  Constant_x_dd_a5fb7 : Constant  Value=x_dd
  Constant_x_ddd_b0e15 : Constant  Value=x_ddd
  Constant_x_ddd_c7c64 : Constant  Value=x_ddd
  Constant_x_ddd_e3c4c : Constant  Value=x_ddd
  Constant_x_l_62f5c : Constant  Value=x_l
  Constant_x_l_68c3a : Constant  Value=x_l
  Constant_x_l_bcbf6 : Constant  Value=x_l
  Divide_022f9 : Product  Inputs=*/
  Divide_4c064 : Product  Inputs=*/
  Divide_733dd : Product  Inputs=*/
  Divide_d5fc9 : Product  Inputs=*/
  MathFunc_cos_3f09e : Trigonometry  Operator=cos
  MathFunc_sin_982c7 : Trigonometry
  Product_088d5 : Product
  Product_1f9cf : Product
  Product_2f3af : Product
  Product_55c3a : Product
  Product_6186a : Product
  Product_62ba0 : Product
  Product_6de55 : Product
  Product_7138e : Product
  Product_7bccc : Product
  Product_9eab9 : Product
  Product_c23ce : Product
  Product_cd532 : Product
  Subtract_33045 : Sum  Inputs=+-
  Subtract_367ef : Sum  Inputs=+-
  Subtract_3d762 : Sum  Inputs=+-
  Subtract_b4479 : Sum  Inputs=+-
  Subtract_c0b64 : Sum  Inputs=+-
  Subtract_d4056 : Sum  Inputs=+-
  Subtract_d9075 : Sum  Inputs=+-
  Blockout_d_psi_d_SG_D_3_27069 : Outport
  wires:
  Constant_-1_4ed88/1 -> Product_cd532/1
  Constant_2.0_62dc7/1 -> Product_088d5/1
  Constant_x_dd_24fcc/1 -> Subtract_33045/1
  State_psi_1d_SG_D_3_2013b/1 -> Product_cd532/2
  Constant_x_dd_079ee/1 -> Subtract_d9075/1
  Constant_pi_2a548/1 -> Product_088d5/2
  Constant_x_ddd_c7c64/1 -> Subtract_33045/2
  Product_cd532/1 -> Product_7bccc/1
  Product_088d5/1 -> Product_55c3a/1
  Subtract_33045/1 -> Product_7bccc/2
  Constant_-2.0_f1148/1 -> Product_c23ce/1
  Constant_x_l_62f5c/1 -> Subtract_d9075/2
  Constant_x_ddd_e3c4c/1 -> Subtract_367ef/1
  Constant_pi_3c9f0/1 -> Product_c23ce/2
  Constant_x_l_68c3a/1 -> Subtract_367ef/2
  Product_62ba0/1 -> Divide_022f9/1
  Product_7bccc/1 -> Divide_4c064/1
  Subtract_d9075/1 -> Divide_4c064/2
  State_psi_fd_SG_D_3_0e180/1 -> Product_6186a/1
  Subtract_367ef/1 -> Product_6186a/2
  Constant_x_dd_a5fb7/1 -> Subtract_b4479/1
  Constant_x_l_bcbf6/1 -> Subtract_b4479/2
  Divide_022f9/1 -> Subtract_3d762/2
  Divide_4c064/1 -> Add_6de8d/1
  Subtract_d4056/1 -> Product_2f3af/2
  State_psi_d_SG_D_3_d393d/1 -> Add_6de8d/2
  Product_6186a/1 -> Divide_733dd/1
  Subtract_b4479/1 -> Divide_733dd/2
  Add_6de8d/1 -> Subtract_d4056/1
  Divide_733dd/1 -> Subtract_d4056/2
  Product_9eab9/1 -> Add_95d2d/2
  Constant_R_a_63c0e/1 -> Product_2f3af/1
  Product_7138e/1 -> Product_6de55/1
  State_theta_SG_D_3_c5e42/1 -> MathFunc_sin_982c7/1
  Product_2f3af/1 -> Divide_d5fc9/1
  Constant_x_ddd_b0e15/1 -> Divide_d5fc9/2
  Input_v_d_SG_D_3_606f6/1 -> Product_1f9cf/1
  State_w_SG_D_3_5916e/1 -> Product_62ba0/2
  MathFunc_sin_982c7/1 -> Product_1f9cf/2
  State_theta_SG_D_3_aedc7/1 -> MathFunc_cos_3f09e/1
  MathFunc_cos_3f09e/1 -> Product_9eab9/2
  Divide_d5fc9/1 -> Subtract_c0b64/1
  Product_1f9cf/1 -> Subtract_c0b64/2
  Input_v_q_SG_D_3_a4294/1 -> Product_9eab9/1
  State_psi_q_SG_D_3_01c82/1 -> Product_62ba0/1
  Constant_f0_8dd7f/1 -> Product_55c3a/2
  Subtract_c0b64/1 -> Add_95d2d/1
  Product_55c3a/1 -> Divide_022f9/2
  Product_c23ce/1 -> Product_7138e/1
  Constant_f0_938aa/1 -> Product_7138e/2
  Add_95d2d/1 -> Subtract_3d762/1
  Subtract_3d762/1 -> Product_6de55/2
  Product_6de55/1 -> Blockout_d_psi_d_SG_D_3_27069/1

== system case5/SG_D_3/d_psi_fd_SG_D_3_block ==
  note: d_psi_fd_SG_D_3 in case5
      | $-\frac{\psi _{\mathrm{fd},\mathrm{SG},D,3}-E_{\mathrm{fd},\mathrm{SG},D,3}+\left(x_{d}-x_{\mathrm{dd}}\right)\,\left(\frac{\frac{\psi _{\mathrm{1d},\mathrm{SG},D,3}\,\left(x_{\mathrm{dd}}-x_{\mathrm{ddd}}\right)}{x_{\mathrm{dd}}-x_{l}}-\psi _{d,\mathrm{SG},D,3}+\frac{\psi _{\mathrm{fd},\mathrm{SG},D,3}\,\left(x_{\mathrm{ddd}}-x_{l}\right)}{x_{\mathrm{dd}}-x_{l}}}{x_{\mathrm{ddd}}}-\frac{\left(x_{\mathrm{dd}}-x_{\mathrm{ddd}}\right)\,\left(\psi _{\mathrm{1d},\mathrm{SG},D,3}-\psi _{\mathrm{fd},\mathrm{SG},D,3}+\frac{\left(x_{\mathrm{dd}}-x_{l}\right)\,\left(\frac{\psi _{\mathrm{1d},\mathrm{SG},D,3}\,\left(x_{\mathrm{dd}}-x_{\mathrm{ddd}}\right)}{x_{\mathrm{dd}}-x_{l}}-\psi _{d,\mathrm{SG},D,3}+\frac{\psi _{\mathrm{fd},\mathrm{SG},D,3}\,\left(x_{\mathrm{ddd}}-x_{l}\right)}{x_{\mathrm{dd}}-x_{l}}\right)}{x_{\mathrm{ddd}}}\right)}{{\left(x_{\mathrm{dd}}-x_{l}\right)}^2}\right)}{T_{\mathrm{dd}}}$
      | Automatically generated on 2025-10-31 19:12:28 .
  State_E_fd_SG_D_3_c498c : Inport
  State_psi_fd_SG_D_3_7ac4b : Inport  Port=2
  State_psi_1d_SG_D_3_a842a : Inport  Port=3
  State_psi_fd_SG_D_3_12a65 : Inport  Port=4
  State_psi_1d_SG_D_3_8aaf0 : Inport  Port=5
  State_psi_d_SG_D_3_99e22 : Inport  Port=6
  State_psi_fd_SG_D_3_2014a : Inport  Port=7
  State_psi_1d_SG_D_3_7f19e : Inport  Port=8
  State_psi_d_SG_D_3_9a2c9 : Inport  Port=9
  State_psi_fd_SG_D_3_0d84b : Inport  Port=10
  Add_cdcd2 : Sum
  Add_d17ea : Sum
  Constant_-1_43d4e : Constant  Value=-1
  Constant_-1_7936c : Constant  Value=-1
  Constant_-1_8ab3d : Constant  Value=-1
  Constant_2.0_99b29 : Constant  Value=2.0
  Constant_T_dd_e7683 : Constant  Value=T_dd
  Constant_x_d_cd02a : Constant  Value=x_d
  Constant_x_dd_1253c : Constant  Value=x_dd
  Constant_x_dd_204e5 : Constant  Value=x_dd
  Constant_x_dd_2b535 : Constant  Value=x_dd
  Constant_x_dd_3b808 : Constant  Value=x_dd
  Constant_x_dd_449cf : Constant  Value=x_dd
  Constant_x_dd_5a5d5 : Constant  Value=x_dd
  Constant_x_dd_6dfdb : Constant  Value=x_dd
  Constant_x_dd_82733 : Constant  Value=x_dd
  Constant_x_dd_c6f8c : Constant  Value=x_dd
  Constant_x_dd_f2f91 : Constant  Value=x_dd
  Constant_x_ddd_2f015 : Constant  Value=x_ddd
  Constant_x_ddd_3ce41 : Constant  Value=x_ddd
  Constant_x_ddd_3dc72 : Constant  Value=x_ddd
  Constant_x_ddd_51ac8 : Constant  Value=x_ddd
  Constant_x_ddd_b558c : Constant  Value=x_ddd
  Constant_x_ddd_b7eb1 : Constant  Value=x_ddd
  Constant_x_ddd_efcc5 : Constant  Value=x_ddd
  Constant_x_l_02814 : Constant  Value=x_l
  Constant_x_l_2c133 : Constant  Value=x_l
  Constant_x_l_43e93 : Constant  Value=x_l
  Constant_x_l_53b6c : Constant  Value=x_l
  Constant_x_l_56ab0 : Constant  Value=x_l
  Constant_x_l_a229a : Constant  Value=x_l
  Constant_x_l_c9362 : Constant  Value=x_l
  Constant_x_l_f62ee : Constant  Value=x_l
  Divide_0c2d4 : Product  Inputs=*/
  Divide_25e11 : Product  Inputs=*/
  Divide_43ea8 : Product  Inputs=*/
  Divide_51413 : Product  Inputs=*/
  Divide_7ebe6 : Product  Inputs=*/
  Divide_8691a : Product  Inputs=*/
  Divide_9eef9 : Product  Inputs=*/
  Divide_a9652 : Product  Inputs=*/
  Power_da97a : Math  Operator=pow
  Product_0ac0f : Product
  Product_2a81f : Product
  Product_2d84c : Product
  Product_38044 : Product
  Product_3805b : Product
  Product_4f8e7 : Product
  Product_8e4e8 : Product
  Product_9974c : Product
  Product_c8da2 : Product
  Product_dda12 : Product
  Subtract_0a919 : Sum  Inputs=+-
  Subtract_1efb7 : Sum  Inputs=+-
  Subtract_231f5 : Sum  Inputs=+-
  Subtract_23451 : Sum  Inputs=+-
  Subtract_2ce9c : Sum  Inputs=+-
  Subtract_4debe : Sum  Inputs=+-
  Subtract_53399 : Sum  Inputs=+-
  Subtract_58075 : Sum  Inputs=+-
  Subtract_7359c : Sum  Inputs=+-
  Subtract_8a0af : Sum  Inputs=+-
  Subtract_8e2c9 : Sum  Inputs=+-
  Subtract_aecaf : Sum  Inputs=+-
  Subtract_c2152 : Sum  Inputs=+-
  Subtract_df829 : Sum  Inputs=+-
  Subtract_e9a95 : Sum  Inputs=+-
  Subtract_ef4ab : Sum  Inputs=+-
  Subtract_f2c1e : Sum  Inputs=+-
  Subtract_f8338 : Sum  Inputs=+-
  Subtract_f95b8 : Sum  Inputs=+-
  Blockout_d_psi_fd_SG_D_3_9596e : Outport
  wires:
  Product_9974c/1 -> Divide_9eef9/1
  Constant_-1_43d4e/1 -> Product_c8da2/1
  Subtract_1efb7/1 -> Product_4f8e7/2
  State_psi_1d_SG_D_3_8aaf0/1 -> Product_c8da2/2
  Constant_x_l_56ab0/1 -> Subtract_7359c/2
  Constant_x_dd_c6f8c/1 -> Subtract_1efb7/1
  Constant_x_ddd_3ce41/1 -> Subtract_1efb7/2
  Product_c8da2/1 -> Product_4f8e7/1
  Constant_x_dd_204e5/1 -> Subtract_f8338/1
  Constant_x_l_02814/1 -> Subtract_f8338/2
  Constant_x_ddd_b7eb1/1 -> Subtract_2ce9c/2
  Constant_x_ddd_b558c/1 -> Subtract_aecaf/1
  Constant_x_l_a229a/1 -> Subtract_aecaf/2
  Product_2d84c/1 -> Product_dda12/1
  Product_4f8e7/1 -> Divide_0c2d4/1
  Subtract_f8338/1 -> Divide_0c2d4/2
  State_psi_fd_SG_D_3_2014a/1 -> Product_38044/1
  Constant_x_ddd_3dc72/1 -> Subtract_7359c/1
  Subtract_aecaf/1 -> Product_38044/2
  Constant_x_dd_2b535/1 -> Subtract_4debe/1
  Constant_-1_8ab3d/1 -> Product_2d84c/1
  Constant_x_l_43e93/1 -> Subtract_4debe/2
  Product_dda12/1 -> Divide_25e11/1
  Divide_0c2d4/1 -> Add_cdcd2/1
  Product_3805b/1 -> Divide_8691a/1
  State_psi_d_SG_D_3_99e22/1 -> Add_cdcd2/2
  State_psi_fd_SG_D_3_0d84b/1 -> Product_3805b/1
  Product_38044/1 -> Divide_7ebe6/1
  Constant_x_dd_3b808/1 -> Subtract_53399/1
  Subtract_4debe/1 -> Divide_7ebe6/2
  Constant_x_l_2c133/1 -> Subtract_df829/2
  Constant_x_dd_1253c/1 -> Subtract_58075/1
  Subtract_e9a95/1 -> Product_8e4e8/2
  Constant_x_l_c9362/1 -> Subtract_58075/2
  Divide_25e11/1 -> Add_d17ea/1
  Constant_x_ddd_51ac8/1 -> Divide_9eef9/2
  Add_cdcd2/1 -> Subtract_231f5/1
  Divide_7ebe6/1 -> Subtract_231f5/2
  State_psi_1d_SG_D_3_7f19e/1 -> Product_2d84c/2
  Constant_x_l_f62ee/1 -> Subtract_53399/2
  Constant_x_dd_f2f91/1 -> Subtract_2ce9c/1
  Subtract_58075/1 -> Product_9974c/1
  Add_d17ea/1 -> Subtract_c2152/1
  Subtract_231f5/1 -> Product_9974c/2
  Subtract_2ce9c/1 -> Product_dda12/2
  Constant_x_dd_449cf/1 -> Subtract_8a0af/1
  Constant_x_l_53b6c/1 -> Subtract_8a0af/2
  Subtract_7359c/1 -> Product_3805b/2
  Constant_x_dd_6dfdb/1 -> Subtract_e9a95/1
  Constant_x_ddd_efcc5/1 -> Subtract_e9a95/2
  Product_8e4e8/1 -> Product_2a81f/1
  State_psi_1d_SG_D_3_a842a/1 -> Subtract_23451/1
  Subtract_8a0af/1 -> Divide_25e11/2
  State_psi_fd_SG_D_3_12a65/1 -> Subtract_23451/2
  Constant_-1_7936c/1 -> Product_8e4e8/1
  Subtract_23451/1 -> Subtract_f2c1e/1
  Divide_9eef9/1 -> Subtract_f2c1e/2
  Constant_x_dd_5a5d5/1 -> Subtract_df829/1
  Divide_8691a/1 -> Subtract_c2152/2
  State_psi_d_SG_D_3_9a2c9/1 -> Add_d17ea/2
  Subtract_53399/1 -> Divide_8691a/2
  Subtract_f2c1e/1 -> Product_2a81f/2
  Subtract_df829/1 -> Power_da97a/1
  Constant_2.0_99b29/1 -> Power_da97a/2
  Product_2a81f/1 -> Divide_43ea8/1
  Subtract_8e2c9/1 -> Product_0ac0f/2
  Power_da97a/1 -> Divide_43ea8/2
  Subtract_c2152/1 -> Divide_a9652/1
  Constant_x_ddd_2f015/1 -> Divide_a9652/2
  Constant_x_d_cd02a/1 -> Subtract_0a919/1
  Constant_x_dd_82733/1 -> Subtract_0a919/2
  Divide_43ea8/1 -> Subtract_8e2c9/1
  Divide_a9652/1 -> Subtract_8e2c9/2
  State_E_fd_SG_D_3_c498c/1 -> Subtract_ef4ab/1
  State_psi_fd_SG_D_3_7ac4b/1 -> Subtract_ef4ab/2
  Subtract_0a919/1 -> Product_0ac0f/1
  Subtract_ef4ab/1 -> Subtract_f95b8/1
  Product_0ac0f/1 -> Subtract_f95b8/2
  Subtract_f95b8/1 -> Divide_51413/1
  Constant_T_dd_e7683/1 -> Divide_51413/2
  Divide_51413/1 -> Blockout_d_psi_fd_SG_D_3_9596e/1
